simulink model "simpSimuRoboToGoRegelKaskade"  (R2019b)
settings: Solver=FixedStepDiscrete  StartTime=0.0  StopTime=100  FixedStep=0.1  RelTol=1e-3  EnableMultiTasking=on
libraries: simulink_extras x2, simulink x2, fahrradDiskr x1
settings Model: Creator=pic  LastModifiedBy=mackst
settings SolverCC: ZeroCrossAlgorithm=Adaptive
settings DataIOCC: SaveFormat=Array  TimeSaveName=t  OutputSaveName=y
settings OptimizationCC: ExpressionDepthLimit=2147483647  LifeSpan=inf
settings DebuggingCC: UnderspecifiedInitializationDetection=Classic  MergeDetectMultiDrivingBlocksExec=none  SolverPrmCheckMsg=warning  AllowSymbolicDim=off  StateNameClashWarn=warning  SFUnexpectedBacktrackingDiag=warning  SFNoUnconditionalDefaultTransitionDiag=warning  SFExecutionAtInitializationDiag=none  ArithmeticOperatorsInVariantConditions=warning
settings HardwareCC: ProdBitPerPointer=32  ProdBitPerSizeT=32  ProdBitPerPtrDiffT=32  ProdLargestAtomicFloat=None  ProdIntDivRoundTo=Undefined  ProdEndianess=Unspecified  ProdWordSize=32  ProdHWDeviceType=32-bit Generic
settings ModelReferenceCC: PropagateSignalLabelsOutOfModel=off
settings SFSimCC: SimUseLocalCustomCode=off  CustomCodeUndefinedFunction=UseInterfaceOnly
settings RTWCC: RTWUseLocalCustomCode=off
settings CodeAppCC: StateflowObjectComments=on
settings GRTTargetCC: TargetLangStandard=C89/C90 (ANSI)  CombineOutputUpdateFcns=off  GRTInterface=on
settings ConfigComp: CovMetricSettings=dw  CovSaveCumulativeToWorkspaceVar=on  CovSaveSingleToWorkspaceVar=on  CovExternalEMLEnable=off

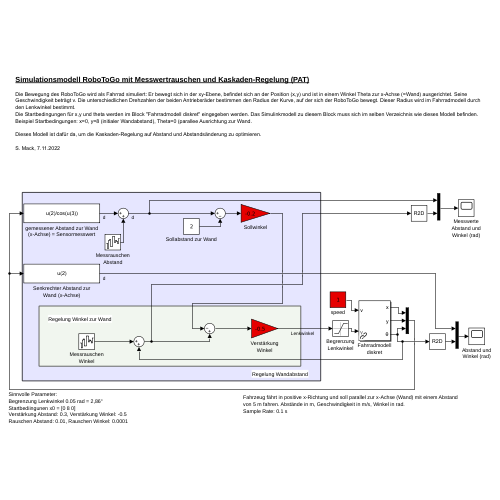
[thumbnail: Simulink's stored preview of the top-level diagram]
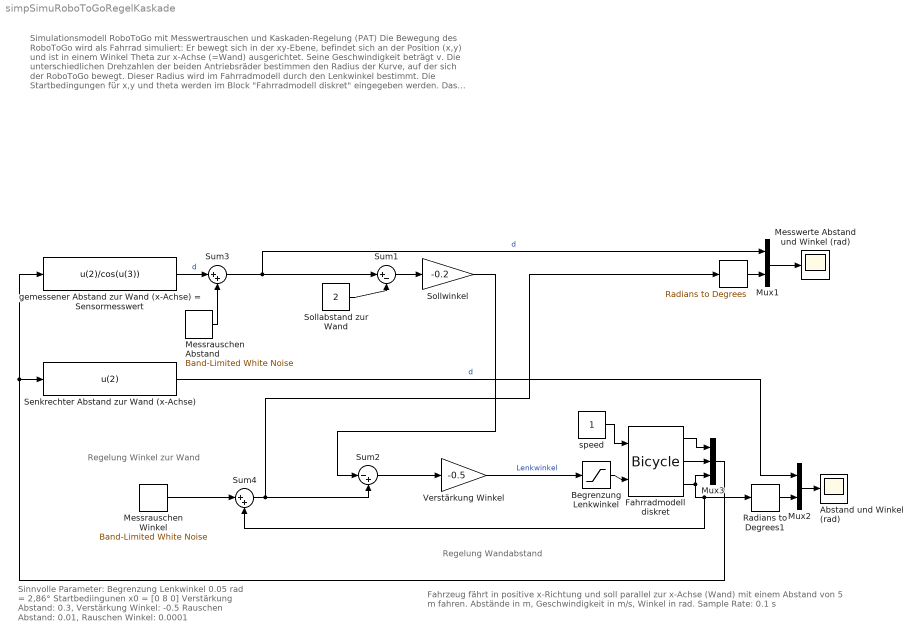
== system simpSimuRoboToGoRegelKaskade ==
  note: Sinnvolle Parameter:
      | Begrenzung Lenkwinkel 0.05 rad = 2,86°
      | Startbediingunen x0 = [0 8 0]
      | Verstärkung Abstand: 0.3, Verstärkung Winkel: -0.5
      | Rauschen Abstand: 0.01, Rauschen Winkel: 0.0001
  note: Regelung Wandabstand
  note: Regelung Winkel zur Wand
  note: Simulationsmodell RoboToGo mit Messwertrauschen und Kaskaden-Regelung (PAT)
      |
      | Die Bewegung des RoboToGo wird als Fahrrad simuliert: Er bewegt sich in der xy-Ebene, befindet sich an der Position (x,y) und ist in einem Winkel Theta zur x-Achse (=Wand) ausgerichtet. Seine Geschwindigkeit beträgt v. Die unterschiedlichen Drehzahlen der beiden Antriebsräder bestimmen den Radius der Kurve, auf der sich der RoboToGo bewegt. Dieser Radius wird im Fahrradmodell durch den Lenkwinkel bestimmt.
      | Die Startbedingungen für x,y und theta werden im Block "Fahrradmodell diskret" eingegeben werden. Das Simulinkmodell zu diesem Block muss sich im selben Verzeichnis wie dieses Modell befinden. Beispiel Startbedingungen: x=0, y=8 (initialer Wandabstand), Theta=0 (parallee Ausrichtung zur Wand.
      |
      | Dieses Modell ist dafür da, um die Kaskaden-Regelung auf Abstand und Abstandsänderung zu optimieren.
      |
      | S. Mack, 7.11.2022
  note: Fahrzeug fährt in positive x-Richtung und soll parallel zur x-Achse (Wand) mit einem Abstand
      | von 5 m fahren. Abstände in m, Geschwindigkeit in m/s, Winkel in rad.
      | Sample Rate: 0.1 s
  " " : simulink_extras/Transformations/Radians to Degrees
  Abstand und Winkel (rad) : Scope
  Begrenzung Lenkwinkel : Saturate  UpperLimit=0.05  LowerLimit=-0.05
  Fahrradmodell diskret : fahrradDiskr/Vehicles/Bicycle  vlim=1  accel=Inf  alim=Inf  steer_rate=Inf  L=1  x0=[0, 8, 0]
  Messrauschen Abstand : simulink/Sources/Band-Limited White Noise  Cov=[0.01]  Ts=0.1  seed=[23341]
  Messrauschen Winkel : simulink/Sources/Band-Limited White Noise  Cov=[0.0001]  Ts=0.1  seed=[23341]
  Messwerte Abstand und Winkel (rad) : Scope
  Mux1 : Mux  Inputs=2
  Mux2 : Mux  Inputs=2
  Mux3 : Mux  Inputs=3
  Radians to Degrees1 : simulink_extras/Transformations/Radians to Degrees
  Senkrechter Abstand zur Wand (x-Achse) : Fcn  Expr=u(2)
  Sollabstand zur Wand : Constant  Value=2  SampleTime=-1
  Sollwinkel : Gain  Gain=-0.2
  Sum1 : Sum  Inputs=|+-
  Sum2 : Sum  Inputs=|-+
  Sum3 : Sum  Inputs=|++
  Sum4 : Sum  Inputs=|++
  Verstärkung Winkel : Gain  Gain=-0.5
  gemessener Abstand zur Wand (x-Achse) = Sensormesswert : Fcn  Expr=u(2)/cos(u(3))
  speed : Constant  VectorParams1D=off  SampleTime=-1
  wires:
  Mux3/1 -> gemessener Abstand zur Wand (x-Achse) = Sensormesswert/1, Senkrechter Abstand zur Wand (x-Achse)/1
  speed/1 -> Fahrradmodell diskret/1
  Verstärkung Winkel/1 -> Begrenzung Lenkwinkel/1  "Lenkwinkel"
  Fahrradmodell diskret/1 -> Mux3/1
  Fahrradmodell diskret/2 -> Mux3/2
  Fahrradmodell diskret/3 -> Sum4/2, Radians to Degrees1/1, Mux3/3
  Sum1/1 -> Sollwinkel/1
  Sollabstand zur Wand/1 -> Sum1/2
  Sum3/1 -> Mux1/1, Sum1/1  "d"
  Senkrechter Abstand zur Wand (x-Achse)/1 -> Mux2/1  "d"
  Sum2/1 -> Verstärkung Winkel/1
  Messrauschen Abstand/1 -> Sum3/2
  gemessener Abstand zur Wand (x-Achse) = Sensormesswert/1 -> Sum3/1  "d"
  Messrauschen Winkel/1 -> Sum4/1
  Sum4/1 -> " "/1, Sum2/2
  Mux2/1 -> Abstand und Winkel (rad)/1
  Mux1/1 -> Messwerte Abstand und Winkel (rad)/1
  " "/1 -> Mux1/2
  Radians to Degrees1/1 -> Mux2/2
  Begrenzung Lenkwinkel/1 -> Fahrradmodell diskret/2
  Sollwinkel/1 -> Sum2/1
